simulink library "libsb2sl"  (Simulink 7.3)
settings: Solver=ode45  SolverMode=SingleTasking  StartTime=0.0  StopTime=10.0  RelTol=1e-3
PostLoadFcn:
  | setsysloc libsb2sl
undefined symbols (not defined in the file): A, Ac, Ad, B, Bc, Bd, C, Cc, Cd, code, const, D, data, Dc, Dd, DiscIntNeverNeededParam, gain, info, k, m, map, no, stat, X0, xd, xi
libraries: simulink3 x17, simulink x5, libsb2sl x3
(part 3 of 3)

== system libsb2sl/DYN/DIntegrator/NthOrder ==
  u : Inport  SampleTime=TS  OutDataType=sfix(16)  OutScaling=2^0
  Demux : Demux  Outputs=[no no*N]
  Gain : Gain  Gain=K  ParameterDataType=sfix(16)  ParameterScaling=2^0  OutDataType=sfix(16)  OutScaling=2^0  SaturateOnIntegerOverflow=on  OutDataTypeStr=Inherit: Same as input  ParamDataTypeStr=Inherit: Same as input
  Integrator : DiscreteIntegrator  InitialCondition=X0  SampleTime=TS  OutDataType=sfix(16)  OutScaling=2^0  ICPrevOutput=DiscIntNeverNeededParam  ICPrevScaledInput=DiscIntNeverNeededParam
  Mux : Mux  Inputs=[no no*N]
  StateMap : Selector  InputPortWidth=no*(1+N)  IndexOptions=Index vector (dialog)  Indices=stateMap  OutputSizes=1
  y : Outport  OutDataType=sfix(16)  OutScaling=2^0
  wires:
  Mux/1 -> StateMap/1
  StateMap/1 -> Demux/1
  Integrator/1 -> Mux/2
  Demux/2 -> Integrator/1
  u/1 -> Mux/1
  Demux/1 -> Gain/1
  Gain/1 -> y/1

== system libsb2sl/DYN/DIntegrator/NthOrder1 ==
  u : Inport  SampleTime=TS  OutDataType=sfix(16)  OutScaling=2^0
  Demux : Demux  Outputs=[no no*N]
  Integrator : DiscreteIntegrator  InitialCondition=X0  SampleTime=TS  OutDataType=sfix(16)  OutScaling=2^0  ICPrevOutput=DiscIntNeverNeededParam  ICPrevScaledInput=DiscIntNeverNeededParam
  Mux : Mux  Inputs=[no no*N]
  StateMap : Selector  InputPortWidth=no*(1+N)  IndexOptions=Index vector (dialog)  Indices=stateMap  OutputSizes=1
  y : Outport  OutDataType=sfix(16)  OutScaling=2^0
  wires:
  u/1 -> Mux/1
  Demux/2 -> Integrator/1
  Integrator/1 -> Mux/2
  StateMap/1 -> Demux/1
  Mux/1 -> StateMap/1
  Demux/1 -> y/1

== system libsb2sl/DYN/DPIDControlLaw/D Term ==
  e : Inport  OutDataType=sfix(16)  OutScaling=2^0
  Enable D Term : EnablePort  StatesWhenEnabling=reset
  Derivative : Gain  Gain=D  ParameterDataType=sfix(16)  ParameterScaling=2^0  OutDataType=sfix(16)  OutScaling=2^0  SaturateOnIntegerOverflow=on  OutDataTypeStr=Inherit: Same as input  ParamDataTypeStr=Inherit: Same as input
  Sum1 : Sum  Inputs=-++  OutDataType=sfix(16)  OutScaling=2^0  SaturateOnIntegerOverflow=on  InputSameDT=on  OutDataTypeStr=Inherit: Same as first input
  TimeConstant2 : Gain  Gain=1/(TAU+TS(1))  ParameterDataType=sfix(16)  ParameterScaling=2^0  OutDataType=sfix(16)  OutScaling=2^0  SaturateOnIntegerOverflow=on  OutDataTypeStr=Inherit: Same as input  ParamDataTypeStr=Inherit: Same as input
  TimeConstant3 : Gain  Gain=TAU  ParameterDataType=sfix(16)  ParameterScaling=2^0  OutDataType=sfix(16)  OutScaling=2^0  SaturateOnIntegerOverflow=on  OutDataTypeStr=Inherit: Same as input  ParamDataTypeStr=Inherit: Same as input
  ed : UnitDelay  SampleTime=TS
  xd : UnitDelay  X0=xd  SampleTime=TS
  u_d : Outport  OutDataType=sfix(16)  OutScaling=2^0
  wires:
  TimeConstant2/1 -> Derivative/1, xd/1
  Derivative/1 -> u_d/1
  xd/1 -> TimeConstant3/1
  Sum1/1 -> TimeConstant2/1
  TimeConstant3/1 -> Sum1/3
  ed/1 -> Sum1/1
  e/1 -> Sum1/2, ed/1

== system libsb2sl/DYN/DPIDControlLaw/I Term ==
  e : Inport  OutDataType=sfix(16)  OutScaling=2^0
  Enable I Term : EnablePort  StatesWhenEnabling=reset
  Integral : Gain  Gain=I  ParameterDataType=sfix(16)  ParameterScaling=2^0  OutDataType=sfix(16)  OutScaling=2^0  SaturateOnIntegerOverflow=on  OutDataTypeStr=Inherit: Same as input  ParamDataTypeStr=Inherit: Same as input
  Sum2 : Sum  OutDataType=sfix(16)  OutScaling=2^0  SaturateOnIntegerOverflow=on  InputSameDT=on  OutDataTypeStr=Inherit: Same as first input
  TimeConstant1 : Gain  Gain=TS(1)  ParameterDataType=sfix(16)  ParameterScaling=2^0  OutDataType=sfix(16)  OutScaling=2^0  SaturateOnIntegerOverflow=on  OutDataTypeStr=Inherit: Same as input  ParamDataTypeStr=Inherit: Same as input
  xi : UnitDelay  X0=xi  SampleTime=TS
  u_i : Outport  OutDataType=sfix(16)  OutScaling=2^0
  wires:
  e/1 -> TimeConstant1/1
  TimeConstant1/1 -> Sum2/1
  xi/1 -> Sum2/2
  Sum2/1 -> xi/1, Integral/1
  Integral/1 -> u_i/1

== system libsb2sl/DYN/DResetIntegrator/1stOrder ==
  u : Inport  SampleTime=TS  OutDataType=sfix(16)  OutScaling=2^0
  new : Inport  Port=2  SampleTime=TS  OutDataType=sfix(16)  OutScaling=2^0
  reset : Inport  Port=3  SampleTime=TS  OutDataType=sfix(16)  OutScaling=2^0
  Gain : Gain  Gain=K  ParameterDataType=sfix(16)  ParameterScaling=2^0  OutDataType=sfix(16)  OutScaling=2^0  SaturateOnIntegerOverflow=on  OutDataTypeStr=Inherit: Same as input  ParamDataTypeStr=Inherit: Same as input
  IC : InitialCondition  Value=X0
  Integrator : DiscreteIntegrator  ExternalReset=rising  InitialConditionSource=external  InitialCondition=X0  SampleTime=TS  OutDataType=sfix(16)  OutScaling=2^0  ICPrevOutput=DiscIntNeverNeededParam  ICPrevScaledInput=DiscIntNeverNeededParam
  y : Outport  OutDataType=sfix(16)  OutScaling=2^0
  wires:
  IC/1 -> Integrator/3
  reset/1 -> Integrator/2
  new/1 -> IC/1
  u/1 -> Integrator/1
  Gain/1 -> y/1
  Integrator/1 -> Gain/1

== system libsb2sl/DYN/DResetIntegrator/1stOrder1 ==
  u : Inport  SampleTime=TS  OutDataType=sfix(16)  OutScaling=2^0
  new : Inport  Port=2  SampleTime=TS  OutDataType=sfix(16)  OutScaling=2^0
  reset : Inport  Port=3  SampleTime=TS  OutDataType=sfix(16)  OutScaling=2^0
  IC : InitialCondition  Value=X0
  Integrator : DiscreteIntegrator  ExternalReset=rising  InitialConditionSource=external  InitialCondition=X0  SampleTime=TS  OutDataType=sfix(16)  OutScaling=2^0  ICPrevOutput=DiscIntNeverNeededParam  ICPrevScaledInput=DiscIntNeverNeededParam
  y : Outport  OutDataType=sfix(16)  OutScaling=2^0
  wires:
  u/1 -> Integrator/1
  new/1 -> IC/1
  reset/1 -> Integrator/2
  IC/1 -> Integrator/3
  Integrator/1 -> y/1

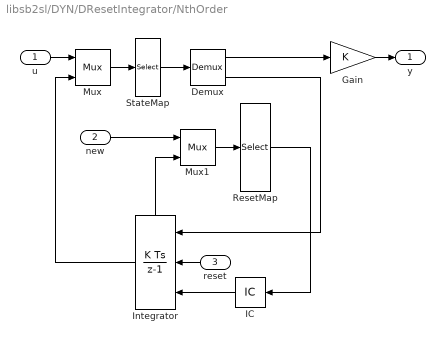
== system libsb2sl/DYN/DResetIntegrator/NthOrder ==
  u : Inport  SampleTime=TS  OutDataType=sfix(16)  OutScaling=2^0
  new : Inport  Port=2  SampleTime=TS  OutDataType=sfix(16)  OutScaling=2^0
  reset : Inport  Port=3  SampleTime=TS  OutDataType=sfix(16)  OutScaling=2^0
  Demux : Demux  Outputs=[no no*N]
  Gain : Gain  Gain=K  ParameterDataType=sfix(16)  ParameterScaling=2^0  OutDataType=sfix(16)  OutScaling=2^0  SaturateOnIntegerOverflow=on  OutDataTypeStr=Inherit: Same as input  ParamDataTypeStr=Inherit: Same as input
  IC : InitialCondition  Value=X0
  Integrator : DiscreteIntegrator  ExternalReset=rising  InitialConditionSource=external  InitialCondition=X0  SampleTime=TS  OutDataType=sfix(16)  OutScaling=2^0  ShowStatePort=on  ICPrevOutput=DiscIntNeverNeededParam  ICPrevScaledInput=DiscIntNeverNeededParam
  Mux : Mux  Inputs=[no no*N]
  Mux1 : Mux  Inputs=[NR N]*no
  ResetMap : Selector  InputPortWidth=(NR+N)*no  IndexOptions=Index vector (dialog)  Indices=resetMap  OutputSizes=1
  StateMap : Selector  InputPortWidth=no*(1+N)  IndexOptions=Index vector (dialog)  Indices=stateMap  OutputSizes=1
  y : Outport  OutDataType=sfix(16)  OutScaling=2^0
  wires:
  Demux/1 -> Gain/1
  u/1 -> Mux/1
  StateMap/1 -> Demux/1
  Mux/1 -> StateMap/1
  IC/1 -> Integrator/3
  Integrator/1 -> Mux/2
  reset/1 -> Integrator/2
  ResetMap/1 -> IC/1
  new/1 -> Mux1/1
  Mux1/1 -> ResetMap/1
  Integrator/State -> Mux1/2
  Gain/1 -> y/1
  Demux/2 -> Integrator/1

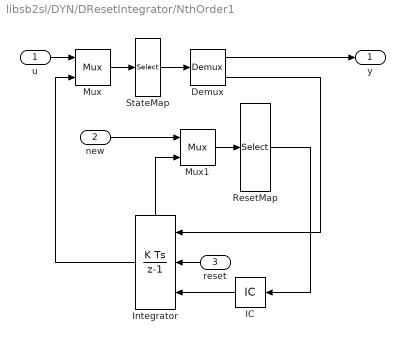
== system libsb2sl/DYN/DResetIntegrator/NthOrder1 ==
  u : Inport  SampleTime=TS  OutDataType=sfix(16)  OutScaling=2^0
  new : Inport  Port=2  SampleTime=TS  OutDataType=sfix(16)  OutScaling=2^0
  reset : Inport  Port=3  SampleTime=TS  OutDataType=sfix(16)  OutScaling=2^0
  Demux : Demux  Outputs=[no no*N]
  IC : InitialCondition  Value=X0
  Integrator : DiscreteIntegrator  ExternalReset=rising  InitialConditionSource=external  InitialCondition=X0  SampleTime=TS  OutDataType=sfix(16)  OutScaling=2^0  ShowStatePort=on  ICPrevOutput=DiscIntNeverNeededParam  ICPrevScaledInput=DiscIntNeverNeededParam
  Mux : Mux  Inputs=[no no*N]
  Mux1 : Mux  Inputs=[NR N]*no
  ResetMap : Selector  InputPortWidth=(NR+N)*no  IndexOptions=Index vector (dialog)  Indices=resetMap  OutputSizes=1
  StateMap : Selector  InputPortWidth=no*(1+N)  IndexOptions=Index vector (dialog)  Indices=stateMap  OutputSizes=1
  y : Outport  OutDataType=sfix(16)  OutScaling=2^0
  wires:
  Demux/2 -> Integrator/1
  Integrator/State -> Mux1/2
  Mux1/1 -> ResetMap/1
  new/1 -> Mux1/1
  ResetMap/1 -> IC/1
  reset/1 -> Integrator/2
  Integrator/1 -> Mux/2
  IC/1 -> Integrator/3
  Mux/1 -> StateMap/1
  StateMap/1 -> Demux/1
  u/1 -> Mux/1
  Demux/1 -> y/1
